simulink model "sampleModel2"  (R2021b)
settings: Solver=VariableStepAuto  StartTime=0.0  StopTime=10.0  RelTol=1e-3
undefined symbols (not defined in the file or in its folder): DiscIntNeverNeededParam, Newton, Raphson
libraries: simulink x12, slpidlib x1
settings Model: Creator=user  LastModifiedBy=user

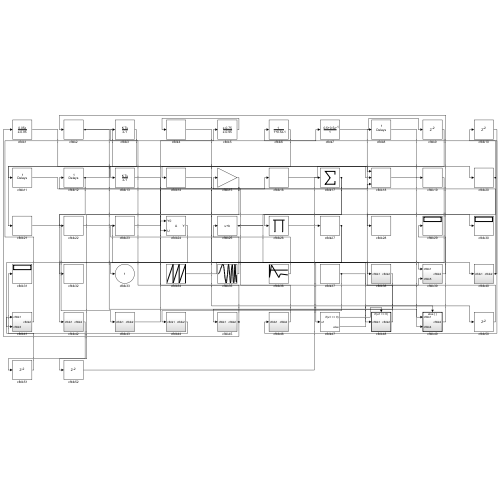
[thumbnail: Simulink's stored preview of the top-level diagram]
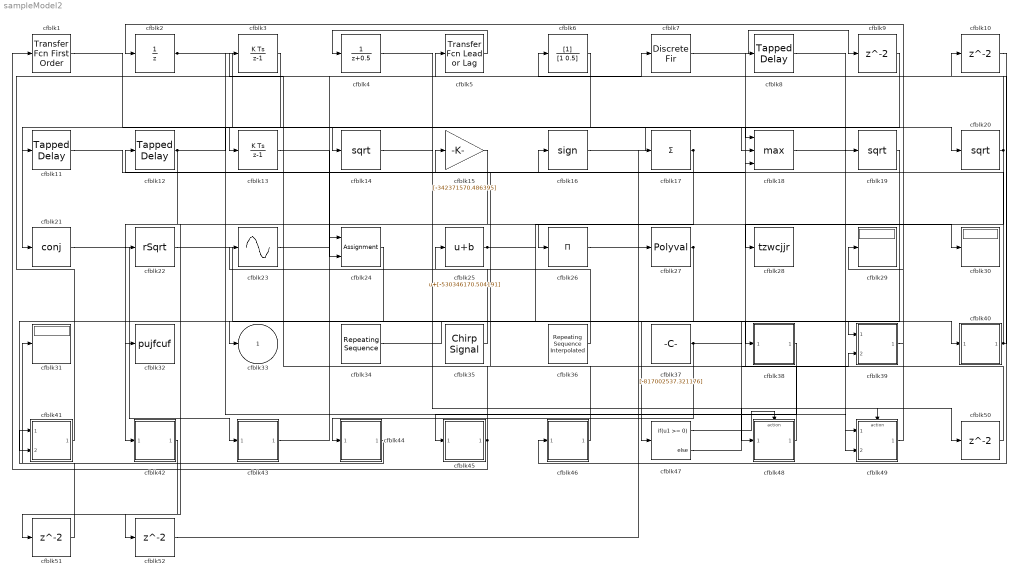
== system sampleModel2 ==
  cfblk1 : simulink/Discrete/Transfer Fcn First Order  PoleZ=0.95  ICPrevOutput=0.0  DoSatur=off
  cfblk{9..10,50..52} (5 alike) : Delay  SampleTime=1
  cfblk11 : simulink/Discrete/Tapped Delay  vinit=0.0  samptime=-1  NumDelays=1  DelayOrder=Oldest  includeCurrent=off
  cfblk12 : simulink/Discrete/Tapped Delay  vinit=0.0  samptime=-1  NumDelays=1  DelayOrder=Oldest  includeCurrent=off
  cfblk13 : DiscreteIntegrator  ICPrevOutput=DiscIntNeverNeededParam  ICPrevScaledInput=DiscIntNeverNeededParam
  cfblk14 : Sqrt  SaturateOnIntegerOverflow=on
  cfblk15 : Gain  Gain=[-342371570.486395]
  cfblk16 : Signum
  cfblk17 : Sum  Inputs=+
  cfblk18 : MinMax  Function=max  Inputs=3
  cfblk19 : Sqrt  SaturateOnIntegerOverflow=on
  cfblk2 : UnitDelay  HasFrameUpgradeWarning=on
  cfblk20 : Sqrt  SaturateOnIntegerOverflow=on
  cfblk21 : Math  Operator=conj  SaturateOnIntegerOverflow=on
  cfblk22 : Sqrt  Operator=rSqrt  AlgorithmType=Newton-Raphson  SaturateOnIntegerOverflow=on
  cfblk23 : Sin  TimeSource=Use external signal  SampleTime=0
  cfblk24 : Assignment  DiagnosticForDimensions=Warning  IndexOptions=Index vector (dialog)  Indices=1  OutputSizes=1
  cfblk25 : Bias  Bias=[-530346170.504191]
  cfblk26 : Product  Inputs=*
  cfblk27 : Polyval  Coefs=[ +2.081618890e-019, -1.441693666e-014, +4.719686976e-010, -8.536869453e-006, +1.621573104e-001, -8.087801117e+001 ]
  cfblk28 : ToWorkspace  VariableName=tzwcjjr  SaveFormat=Timeseries  SampleTime=-1
  cfblk29 : Display
  cfblk3 : DiscreteIntegrator  ICPrevOutput=DiscIntNeverNeededParam  ICPrevScaledInput=DiscIntNeverNeededParam
  cfblk30 : Display
  cfblk31 : Display
  cfblk32 : ToWorkspace  VariableName=pujfcuf  SaveFormat=Timeseries  SampleTime=-1
  cfblk34 : simulink/Sources/Repeating Sequence  rep_seq_t=[0 2]  rep_seq_y=[-223456737.904397, 103557063.914455]
  cfblk35 : simulink/Sources/Chirp Signal  f1=[-542093495.953800]  T=[283881240.798375]  f2=[-31039255.203639]
  cfblk36 : simulink/Sources/Repeating Sequence Interpolated  OutValues=[-696308949.767467, 563863933.176004, -798787355.275157, -411867332.482743, -525253960.588842]  TimeValues=[0 0.1 0.5 0.6 1].'  LookUpMeth=Use Input Below  tsamp=0.01  OutMin=[]  OutMax=[]  OutDataTypeStr=double  OutputDataTypeScalingMode=double  OutDataType=fixdt(0,8)  OutScaling=2^-10
  cfblk37 : Constant  Value=[-817002537.321176]  SampleTime=1
  cfblk38 : Subsystem
  cfblk39 : Subsystem
  cfblk4 : DiscreteTransferFcn  SampleTime=1
  cfblk40 : Subsystem
  cfblk41 : Subsystem
  cfblk42 : Subsystem
  cfblk43 : Subsystem
  cfblk44 : Subsystem
  cfblk45 : Subsystem
  cfblk46 : Subsystem
  cfblk47 : If  IfExpression=u1 >= 0  SampleTime=1
  cfblk48 : Subsystem  TreatAsAtomicUnit=on
  cfblk49 : Subsystem  TreatAsAtomicUnit=on
  cfblk5 : simulink/Discrete/Transfer Fcn Lead or Lag  PoleZ=0.95  ZeroZ=0.75  ICPrevOutput=0.0  ICPrevInput=0.0  DoSatur=off
      settings: SourceProductBaseCode=SL
  cfblk6 : DiscreteFilter  SampleTime=1
  cfblk7 : DiscreteFir  SampleTime=1
  cfblk8 : simulink/Discrete/Tapped Delay  vinit=0.0  samptime=-1  NumDelays=1  DelayOrder=Oldest  includeCurrent=off
  cfblk33 : Outport
  wires:
  cfblk9/1 -> cfblk21/1
  cfblk41/1(cfblk2) -> cfblk5/1
  cfblk7/1 -> cfblk9/1
  cfblk44/1(cfblk2) -> cfblk31/1
  cfblk35/1 -> cfblk25/1
  cfblk48/1(cfblk2) -> cfblk8/1
  cfblk26/1 -> cfblk27/1
  cfblk39/1(cfblk2) -> cfblk2/1
  cfblk4/1 -> cfblk40/1(cfblk1)
  cfblk17/1 -> cfblk26/1, cfblk32/1
  cfblk8/1 -> cfblk19/1
  cfblk1/1 -> cfblk13/1
  cfblk27/1 -> cfblk47/1, cfblk52/1
  cfblk10/1 -> cfblk46/1(cfblk1)
  cfblk38/1(cfblk2) -> cfblk45/1(cfblk1)
  cfblk20/1 -> cfblk28/1, cfblk6/1
  cfblk40/1(cfblk2) -> cfblk12/1, cfblk10/1
  cfblk3/1 -> cfblk11/1
  cfblk34/1 -> cfblk39/1(cfblk1)
  cfblk25/1 -> cfblk38/1(cfblk1), cfblk30/1
  cfblk16/1 -> cfblk18/1
  cfblk15/1 -> cfblk42/1(cfblk1)
  cfblk21/1 -> cfblk43/1(cfblk1)
  cfblk49/1(cfblk2) -> cfblk29/1
  cfblk2/1 -> cfblk18/2, cfblk49/2(cfblk4)
  cfblk24/1 -> cfblk41/2(cfblk3)
  cfblk46/1(cfblk2) -> cfblk15/1
  cfblk23/1 -> cfblk7/1
  cfblk13/1 -> cfblk24/2
  cfblk5/1 -> cfblk4/1
  cfblk11/1 -> cfblk18/3
  cfblk19/1 -> cfblk33/1
  cfblk37/1 -> cfblk44/1(cfblk1), cfblk39/2(cfblk5)
  cfblk12/1 -> cfblk22/1, cfblk20/1
  cfblk18/1 -> cfblk49/1(cfblk1)
  cfblk22/1 -> cfblk48/1(cfblk1)
  cfblk6/1 -> cfblk14/1
  cfblk36/1 -> cfblk23/1
  cfblk45/1(cfblk2) -> cfblk1/1, cfblk3/1
  cfblk43/1(cfblk2) -> cfblk16/1
  cfblk47/1 -> cfblk48/Action
  cfblk47/2 -> cfblk49/Action
  cfblk14/1 -> cfblk50/1
  cfblk50/1 -> cfblk24/1
  cfblk42/1(cfblk2) -> cfblk51/1
  cfblk51/1 -> cfblk41/1(cfblk1)
  cfblk52/1 -> cfblk17/1

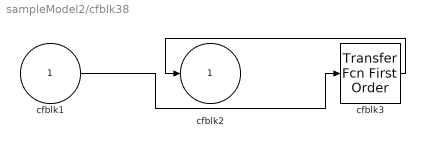
== system sampleModel2/cfblk38 ==
  cfblk1 : Inport
  cfblk3 : simulink/Discrete/Transfer Fcn First Order  PoleZ=0.95  ICPrevOutput=0.0  DoSatur=off
  cfblk2 : Outport
  wires:
  cfblk3/1 -> cfblk2/1
  cfblk1/1 -> cfblk3/1

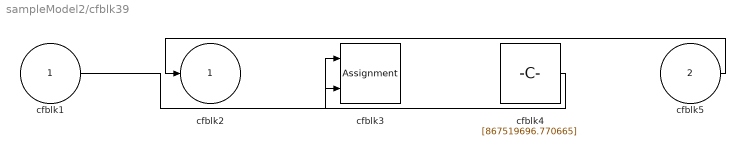
== system sampleModel2/cfblk39 ==
  cfblk1 : Inport
  cfblk5 : Inport  Port=2
  cfblk3 : Assignment  DiagnosticForDimensions=Warning  IndexOptions=Index vector (dialog)  Indices=1  OutputSizes=1
  cfblk4 : Constant  Value=[867519696.770665]  SampleTime=1
  cfblk2 : Outport
  wires:
  cfblk5/1 -> cfblk2/1
  cfblk4/1 -> cfblk3/1
  cfblk1/1 -> cfblk3/2

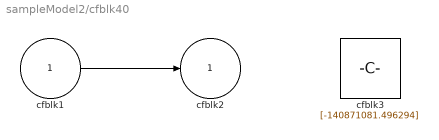
== system sampleModel2/cfblk40 ==
  cfblk1 : Inport
  cfblk3 : Constant  Value=[-140871081.496294]  SampleTime=1
  cfblk2 : Outport
  wires:
  cfblk1/1 -> cfblk2/1

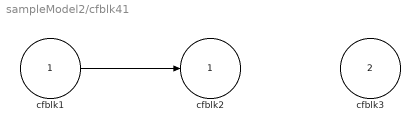
== system sampleModel2/cfblk41 ==
  cfblk1 : Inport
  cfblk3 : Inport  Port=2
  cfblk2 : Outport
  wires:
  cfblk1/1 -> cfblk2/1

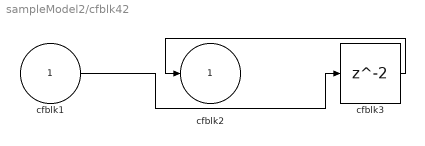
== system sampleModel2/cfblk42 ==
  cfblk1 : Inport
  cfblk3 : Delay  SampleTime=1
  cfblk2 : Outport
  wires:
  cfblk3/1 -> cfblk2/1
  cfblk1/1 -> cfblk3/1

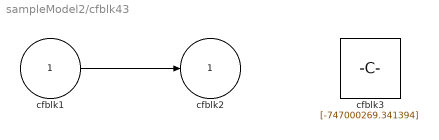
== system sampleModel2/cfblk43 ==
  cfblk1 : Inport
  cfblk3 : Constant  Value=[-747000269.341394]  SampleTime=1
  cfblk2 : Outport
  wires:
  cfblk1/1 -> cfblk2/1

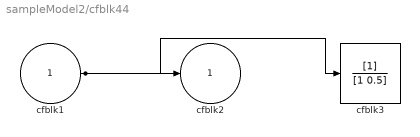
== system sampleModel2/cfblk44 ==
  cfblk1 : Inport
  cfblk3 : DiscreteFilter  SampleTime=1
  cfblk2 : Outport
  wires:
  cfblk1/1 -> cfblk2/1, cfblk3/1

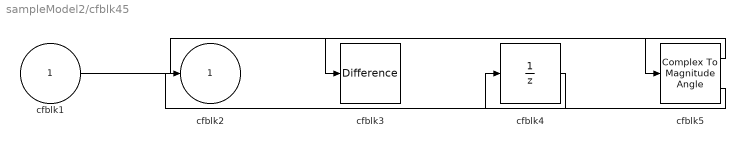
== system sampleModel2/cfblk45 ==
  cfblk1 : Inport
  cfblk3 : simulink/Discrete/Difference  ICPrevInput=0.0  OutMin=[]  OutMax=[]  OutDataTypeStr=Inherit: Inherit via back propagation  OutDataType=fixdt(1, 16)  OutScaling=2^-10  DoSatur=off
  cfblk4 : UnitDelay  HasFrameUpgradeWarning=on
  cfblk5 : ComplexToMagnitudeAngle
  cfblk2 : Outport
  wires:
  cfblk1/1 -> cfblk5/1
  cfblk4/1 -> cfblk2/1
  cfblk5/1 -> cfblk3/1
  cfblk5/2 -> cfblk4/1

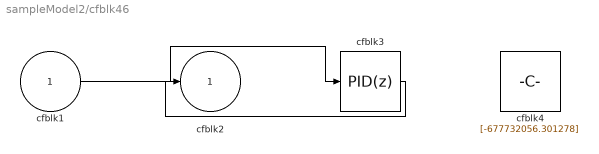
== system sampleModel2/cfblk46 ==
  cfblk1 : Inport
  cfblk3 : slpidlib/PID Controller  Controller=PID  Form=Parallel  TimeDomain=Discrete-time  UseExternalTs=off  SampleTime=1  IntegratorMethod=Forward Euler  FilterMethod=Forward Euler  ControllerParametersSource=internal  P=1  I=1  D=0  UseFilter=on  N=100  TunerSelectOption=Transfer Function Based (PID Tuner App)  InitialConditionSource=internal  InitialConditionForIntegrator=0  InitialConditionForFilter=0  DifferentiatorICPrevScaledInput=0  ExternalReset=none  TrackingMode=off  Kt=1  LimitOutput=off  SatLimitsSource=internal  UpperSaturationLimit=inf  LowerSaturationLimit=-inf  LinearizeAsGain=off  AntiWindupMode=none  Kb=1  POutMin=[]  POutMax=[]  IOutMin=[]  IOutMax=[]  DOutMin=[]  DOutMax=[]  NOutMin=[]  NOutMax=[]  SumOutMin=[]  SumOutMax=[]  SaturationOutMin=[]  SaturationOutMax=[]  PParamMin=[]  PParamMax=[]  IParamMin=[]  IParamMax=[]  DParamMin=[]  DParamMax=[]  NParamMin=[]  NParamMax=[]  KbParamMin=[]  KbParamMax=[]  KtParamMin=[]  KtParamMax=[]  KbOutMin=[]  KbOutMax=[]  KtOutMin=[]  KtOutMax=[]  IntegratorOutMin=[]  IntegratorOutMax=[]  FilterOutMin=[]  FilterOutMax=[]  SumI1OutMin=[]  SumI1OutMax=[]  SumI2OutMin=[]  SumI2OutMax=[]  SumI3OutMin=[]  SumI3OutMax=[]  SumI4OutMin=[]  SumI4OutMax=[]  SumDOutMin=[]  SumDOutMax=[]  DifferentiatorOutMin=[]  DifferentiatorOutMax=[]  FilterDiffOutCoefMin=[]  FilterDiffOutCoefMax=[]  ReciprocalOutMin=[]  ReciprocalOutMax=[]  SumDenOutMin=[]  SumDenOutMax=[]  SumNumOutMin=[]  SumNumOutMax=[]  DivideOutMin=[]  DivideOutMax=[]  UdiffTsProdOutMin=[]  UdiffTsProdOutMax=[]  NTsProdOutMin=[]  NTsProdOutMax=[]  UintegralTsProdOutMin=[]  UintegralTsProdOutMax=[]  UngainTsProdOutMin=[]  UngainTsProdOutMax=[]  IntegratorContinuousStateAttributes=''  IntegratorStateMustResolveToSignalObject=off  IntegratorRTWStateStorageClass=Auto  FilterContinuousStateAttributes=''  FilterStateMustResolveToSignalObject=off  FilterRTWStateStorageClass=Auto  ParallelPVariant=InternalParameters  IdealPVariant=Disabled  IVariant=InternalParameters  DVariant=InternalParameters  IntegratorVariant=Discrete  SatVariant=Disabled  AWVariant=Passthrough  PCopyVariant=Disabled  TRVariant=Disabled  FdbkBlocksVariant=Forward  IdealPFdbkVariant=Disabled  SatFdbkVariant=Disabled  DerivativeFilterVariant=ForwardEulerFilter  NVariant=InternalParameters  NCopyVariant=Disabled  FilterICVariant=InternalICsFilter  IntegratorICVariant=InternalICs  ExternalResetVariant=Disabled  TRSumVariant=Passthrough  SumFdbkVariant=Disabled  SumVariant=Sum_PID  TsampFilterVariant=InternalTs  TsampNgainVariant=Passthrough  TsampIntegralVariant=Passthrough  ExternalSaturationOutDataTypeStr=Inherit: Same as second input
  cfblk4 : Constant  Value=[-677732056.301278]  SampleTime=1
  cfblk2 : Outport
  wires:
  cfblk1/1 -> cfblk3/1
  cfblk3/1 -> cfblk2/1

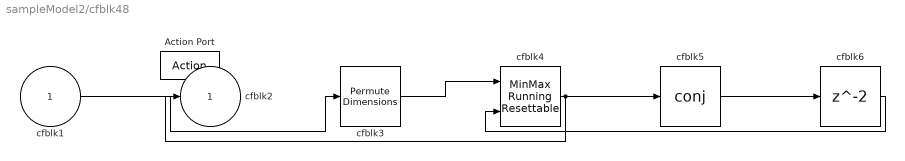
== system sampleModel2/cfblk48 ==
  cfblk1 : Inport
  Action Port : ActionPort  ActionPortLabel=if(u1 >= 0)
  cfblk3 : PermuteDimensions
  cfblk4 : simulink/Math Operations/MinMax Running Resettable  Function=min  vinit=0.0
  cfblk5 : Math  Operator=conj  SaturateOnIntegerOverflow=on
  cfblk6 : Delay
  cfblk2 : Outport
  wires:
  cfblk3/1 -> cfblk4/1
  cfblk1/1 -> cfblk3/1
  cfblk4/1 -> cfblk2/1, cfblk5/1
  cfblk5/1 -> cfblk6/1
  cfblk6/1 -> cfblk4/2

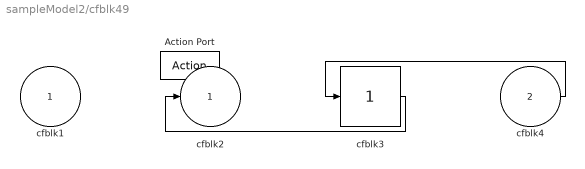
== system sampleModel2/cfblk49 ==
  cfblk1 : Inport
  cfblk4 : Inport  Port=2
  Action Port : ActionPort  ActionPortLabel=else
  cfblk3 : simulink/Math Operations/Slider Gain  gain=1  low=0  high=2
  cfblk2 : Outport
  wires:
  cfblk4/1 -> cfblk3/1
  cfblk3/1 -> cfblk2/1
